simulink library "perturbations"  (R2025b)
settings: Solver=VariableStepAuto  StartTime=0.0  StopTime=10.0  RelTol=1e-3
values from neighbouring files (symbols this model uses):
  g_10 = -29404.8    [lab_7_task_4.m]    (also in project_review.m)
  g_11 = -1450.9    [lab_7_task_4.m]    (also in project_review.m)
  h_11 = 4652.6    [lab_7_task_4.m]    (also in project_review.m = 4652.5)
  I = diag([ix iy iz])    [lab_4_task_1.m]    (also in lab_5_task_1.m; lab_5_task_2.m; lab_6_task_1.m = diag([ ix iy iz ]); lab_6_task_2.m = diag([ ix iy iz ]))
  j = [0.01; 0.05; 0.01;]    [lab_7_task_4.m]    (also in project_review.m)
  mu = astroConstants(13)    [lab_7_task_3.m]    (also in lab_7_task_4.m; project_review.m = 398345.74)
  n_sun = 2*pi / (60*60*24*365)    (= 1.99238499086e-07)    [lab_7_task_1.m]    (also in lab_7_task_2.m; lab_7_task_3.m; lab_7_task_4.m = 1.99102127766e-07; project_review.m = 1.99102127766e-07)
  r_sun = 1.496e8    (= 149600000)    [lab_7_task_1.m]    (also in lab_7_task_2.m; lab_7_task_3.m; lab_7_task_4.m; project_review.m)
libraries: vec_norm x2, SRP x1, matrix_library x1
settings Model: Creator=nicol  LastModifiedBy=nicol

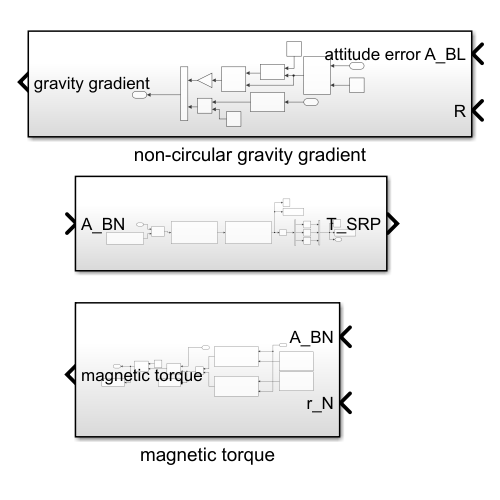
[thumbnail: Simulink's stored preview of the top-level diagram]
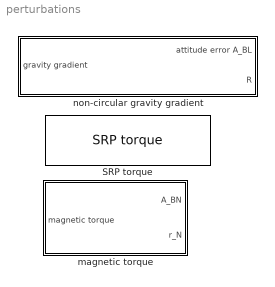
== system perturbations ==
  SRP torque : SRP/SRP torque  SystemSampleTime=-1  VariantActivationTime=update diagram  EmptyChoice=off  PassThrough=off  PassThroughVariantControl=(default)  EmptyChoiceVariantControl=(default)  AllowFlexibleInterface=on  Latency=0  AutoFrameSizeCalculation=off
  magnetic torque : Subsystem
  non-circular gravity gradient : Subsystem
      settings: PortSchema="{\"entries\":[{\"content\":{\"sides\":[{\"content\":{\"connectorIds\":[\"Out1\"]},\"type\":\"ConnectorPlacement.EquallySpacedRectSide\",\"uuid\":\"2a67419a-68c9-4369-a698-e6ac26417455\"},{\"content\":{\"connectorIds\":[\"In1\",\"In2\"],\"side\":\"RIGHT\"},\"type\":\"ConnectorPlacement.EquallySpacedRectSide\",\"uuid\":\"5f3f4c4a-6b79-4b92-8f4c-19ffa36753b2\"},{\"content\":{\"side\":\"TOP\"},\"type\":\"ConnectorPlacement.EquallySpacedRectSide\",\"uuid\":\"22c946b7-ea77-4444-a63c-d5b3d585f671\"}]},\"type\":\"ConnectorPlacement.EquallySpacedConnector\",\"uuid\":\"037c4a72-b28b-418e-a921-9da68dc0cd93\"}],\"packageUris\":[\"http://schema.mathworks.com/mf0/Connector/R2020b\"],\"version\":\"1.0\"}"

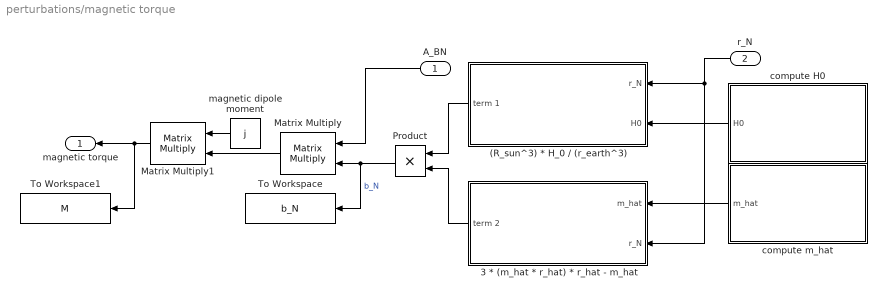
== system perturbations/magnetic torque ==
  A_BN : Inport
  r_N : Inport  Port=2
  (R_sun^3) * H_0 / (r_earth^3) : Subsystem
      settings: PortSchema="{\"entries\":[{\"content\":{\"sides\":[{\"content\":{\"connectorIds\":[\"Out1\"]},\"type\":\"ConnectorPlacement.EquallySpacedRectSide\",\"uuid\":\"bbe988fc-17c4-4719-9870-44bc4a4e76ce\"},{\"content\":{\"connectorIds\":[\"In1\",\"In2\"],\"side\":\"RIGHT\"},\"type\":\"ConnectorPlacement.EquallySpacedRectSide\",\"uuid\":\"575c26dc-e0b7-4e24-b262-40ca05ffcfe5\"},{\"content\":{\"side\":\"TOP\"},\"type\":\"ConnectorPlacement.EquallySpacedRectSide\",\"uuid\":\"0bdf66e4-cddb-4706-9c0a-b23684b15a0a\"}]},\"type\":\"ConnectorPlacement.EquallySpacedConnector\",\"uuid\":\"a70c04a6-2589-454e-b011-fc54f6acc766\"}],\"packageUris\":[\"http://schema.mathworks.com/mf0/Connector/R2020b\"],\"version\":\"1.0\"}"
  3 * (m_hat * r_hat) * r_hat - m_hat : Subsystem
  Matrix Multiply : Product  Multiplication=Matrix(*)
  Matrix Multiply1 : Product  Multiplication=Matrix(*)
  Product : Product
  To Workspace : ToWorkspace  VariableName=b_N  SaveFormat=Timeseries  SampleTime=-1
  To Workspace1 : ToWorkspace  VariableName=M  SaveFormat=Timeseries  SampleTime=-1
  compute H0 : Subsystem
      settings: PortSchema="{\"entries\":[{\"content\":{\"sides\":[{\"content\":{\"connectorIds\":[\"Out1\"]},\"type\":\"ConnectorPlacement.EquallySpacedRectSide\",\"uuid\":\"69538ac4-798d-499e-8a01-9dbb1ae91e13\"},{\"content\":{\"side\":\"RIGHT\"},\"type\":\"ConnectorPlacement.EquallySpacedRectSide\",\"uuid\":\"e472a16b-e756-43b0-a684-24a7beecf6b1\"},{\"content\":{\"side\":\"TOP\"},\"type\":\"ConnectorPlacement.EquallySpacedRectSide\",\"uuid\":\"c0da2b73-1d3e-4f5f-b1be-bce0e733f90d\"}]},\"type\":\"ConnectorPlacement.EquallySpacedConnector\",\"uuid\":\"edf54bcc-843b-4ee1-a337-02c9fdc591b1\"}],\"packageUris\":[\"http://schema.mathworks.com/mf0/Connector/R2020b\"],\"version\":\"1.0\"}"
  compute m_hat : Subsystem
      settings: PortSchema="{\"entries\":[{\"content\":{\"sides\":[{\"content\":{\"connectorIds\":[\"Out1\"]},\"type\":\"ConnectorPlacement.EquallySpacedRectSide\",\"uuid\":\"69538ac4-798d-499e-8a01-9dbb1ae91e13\"},{\"content\":{\"side\":\"RIGHT\"},\"type\":\"ConnectorPlacement.EquallySpacedRectSide\",\"uuid\":\"e472a16b-e756-43b0-a684-24a7beecf6b1\"},{\"content\":{\"side\":\"TOP\"},\"type\":\"ConnectorPlacement.EquallySpacedRectSide\",\"uuid\":\"c0da2b73-1d3e-4f5f-b1be-bce0e733f90d\"}]},\"type\":\"ConnectorPlacement.EquallySpacedConnector\",\"uuid\":\"edf54bcc-843b-4ee1-a337-02c9fdc591b1\"}],\"packageUris\":[\"http://schema.mathworks.com/mf0/Connector/R2020b\"],\"version\":\"1.0\"}"
  magnetic dipole moment : Constant  Value=j
  magnetic torque : Outport
  wires:
  A_BN/1 -> Matrix Multiply/1
  Matrix Multiply1/1 -> magnetic torque/1, To Workspace1/1
  3 * (m_hat * r_hat) * r_hat - m_hat/1(term 2) -> Product/2
  (R_sun^3) * H_0 / (r_earth^3)/1(term 1) -> Product/1
  compute m_hat/1(m_hat) -> 3 * (m_hat * r_hat) * r_hat - m_hat/1(m_hat)
  magnetic dipole moment/1 -> Matrix Multiply1/1
  Product/1 -> To Workspace/1, Matrix Multiply/2  "b_N"
  Matrix Multiply/1 -> Matrix Multiply1/2
  compute H0/1(H0) -> (R_sun^3) * H_0 / (r_earth^3)/2(H0)
  r_N/1 -> 3 * (m_hat * r_hat) * r_hat - m_hat/2(r_N), (R_sun^3) * H_0 / (r_earth^3)/1(r_N)

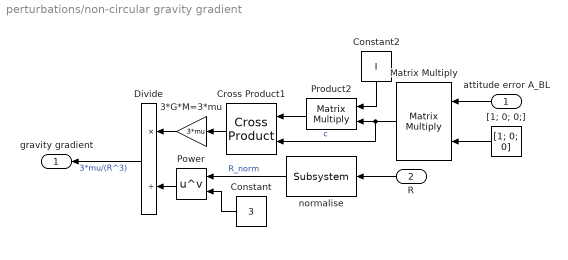
== system perturbations/non-circular gravity gradient ==
  attitude error A_BL : Inport
  R : Inport  Port=2
  3*G*M=3*mu : Gain  Gain=3*mu
  Constant : Constant  Value=3
  Constant2 : Constant  Value=I
  Cross Product1 : matrix_library/Cross Product
  Divide : Product  Inputs=*/
  Matrix Multiply : Product  Multiplication=Matrix(*)
  Power : Math  Operator=pow
  Product2 : Product  Multiplication=Matrix(*)
  "[1; 0; 0;]" : Constant  Value=[1; 0; 0]
  normalise : vec_norm/Subsystem  SystemSampleTime=-1  VariantActivationTime=update diagram  EmptyChoice=off  PassThrough=off  PassThroughVariantControl=(default)  EmptyChoiceVariantControl=(default)  AllowFlexibleInterface=on  Latency=0  AutoFrameSizeCalculation=off
  gravity gradient : Outport
  wires:
  normalise/1 -> Power/1  "R_norm"
  Power/1 -> Divide/2
  Constant/1 -> Power/2
  R/1 -> normalise/1
  Divide/1 -> gravity gradient/1  "3*mu/(R^3)"
  3*G*M=3*mu/1 -> Divide/1
  "[1; 0; 0;]"/1 -> Matrix Multiply/2
  Product2/1 -> Cross Product1/1
  Cross Product1/1 -> 3*G*M=3*mu/1
  Constant2/1 -> Product2/1
  attitude error A_BL/1 -> Matrix Multiply/1
  Matrix Multiply/1 -> Product2/2, Cross Product1/2  "c"

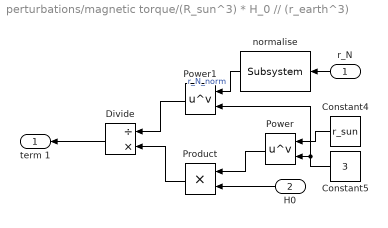
== system perturbations/magnetic torque/(R_sun^3) * H_0 // (r_earth^3) ==
  r_N : Inport
  H0 : Inport  Port=2
  Constant4 : Constant  Value=r_sun
  Constant5 : Constant  Value=3
  Divide : Product  Inputs=/*
  Power : Math  Operator=pow
  Power1 : Math  Operator=pow
  Product : Product
  normalise : vec_norm/Subsystem  SystemSampleTime=-1  VariantActivationTime=update diagram  EmptyChoice=off  PassThrough=off  PassThroughVariantControl=(default)  EmptyChoiceVariantControl=(default)  AllowFlexibleInterface=on  Latency=0  AutoFrameSizeCalculation=off
  term 1 : Outport
  wires:
  normalise/1 -> Power1/1  "r_N_norm"
  Product/1 -> Divide/2
  r_N/1 -> normalise/1
  H0/1 -> Product/2
  Divide/1 -> term 1/1
  Power1/1 -> Divide/1
  Constant5/1 -> Power/2, Power1/2
  Constant4/1 -> Power/1
  Power/1 -> Product/1

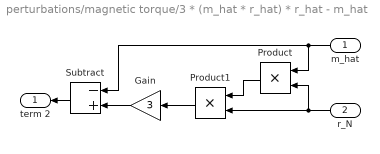
== system perturbations/magnetic torque/3 * (m_hat * r_hat) * r_hat - m_hat ==
  m_hat : Inport
  r_N : Inport  Port=2
  Gain : Gain  Gain=3
  Product : Product
  Product1 : Product
  Subtract : Sum  Inputs=-+
  term 2 : Outport
  wires:
  Gain/1 -> Subtract/2
  Product1/1 -> Gain/1
  Product/1 -> Product1/1
  m_hat/1 -> Product/1, Subtract/1
  Subtract/1 -> term 2/1
  r_N/1 -> Product1/2, Product/2

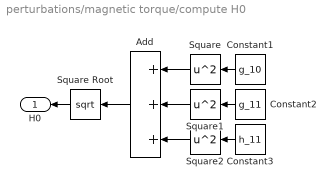
== system perturbations/magnetic torque/compute H0 ==
  Add : Sum  Inputs=+++
  Constant1 : Constant  Value=g_10
  Constant2 : Constant  Value=g_11
  Constant3 : Constant  Value=h_11
  Square : Math  Operator=square
  Square Root : Sqrt
  Square1 : Math  Operator=square
  Square2 : Math  Operator=square
  H0 : Outport
  wires:
  Square/1 -> Add/1
  Square Root/1 -> H0/1
  Add/1 -> Square Root/1
  Square1/1 -> Add/2
  Square2/1 -> Add/3
  Constant3/1 -> Square2/1
  Constant1/1 -> Square/1
  Constant2/1 -> Square1/1

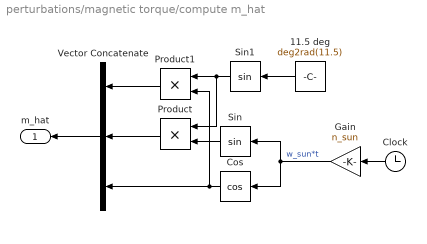
== system perturbations/magnetic torque/compute m_hat ==
  11.5 deg : Constant  Value=deg2rad(11.5)
  Clock : Clock
  Cos : Trigonometry  Operator=cos
  Gain : Gain  Gain=n_sun
  Product : Product
  Product1 : Product
  Sin : Trigonometry
  Sin1 : Trigonometry
  Vector Concatenate : Concatenate  NumInputs=3
  m_hat : Outport
  wires:
  Vector Concatenate/1 -> m_hat/1
  Sin/1 -> Product/2
  Clock/1 -> Gain/1
  Product/1 -> Vector Concatenate/2
  11.5 deg/1 -> Sin1/1
  Sin1/1 -> Product1/1, Product/1
  Gain/1 -> Sin/1, Cos/1  "w_sun*t"
  Cos/1 -> Vector Concatenate/3, Product1/2
  Product1/1 -> Vector Concatenate/1
